simulink model "W2_Problem_4"  (R2020a)
settings: Solver=ode45  StartTime=0.0  StopTime=10.0  RelTol=1e-3
values from neighbouring files (symbols this model uses):
  b = 3.5077E-6    (= 3.5077e-06)    [W2_P4.m]    (also in W2_P4_DD.sldd = 3.5077E-6)
  J = 3.2284E-6    (= 3.2284e-06)    [W2_P4.m]    (also in W2_P4_DD.sldd = 3.2284E-6)
  K = 0.0274    [W2_P4.m]    (also in W2_P4_DD.sldd)
  Kd = Kd + 0.1    (= 0.15)    [W2_P4.m]    (also in W2_P4_DD.sldd = 0.44999999999999996)
  Ki = 500    [W2_P4.m]    (also in W2_P4_DD.sldd = 100.0)
  Kp = 21    [W2_P4.m]    (also in W2_P4_DD.sldd = 21.0)
  L = 2.75E-6    (= 2.75e-06)    [W2_P4.m]    (also in W2_P4_DD.sldd = 2.75E-6)
  R = 4    [W2_P4.m]    (also in W2_P4_DD.sldd = 4.0)
settings Model: Creator=user  LastModifiedBy=user

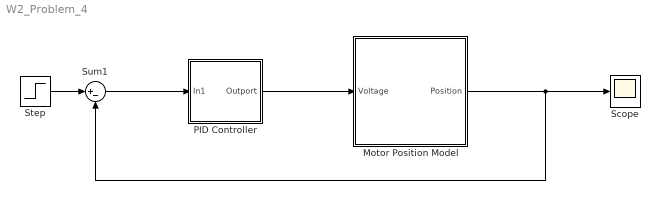
== system W2_Problem_4 ==
  Motor Position Model : Subsystem
  PID Controller : Subsystem
  Scope : Scope
  Step : Step  SampleTime=0
  Sum1 : Sum  Inputs=|+-
  wires:
  PID Controller/1(Outport) -> Motor Position Model/1(Voltage)
  Motor Position Model/1(Position) -> Scope/1, Sum1/2
  Sum1/1 -> PID Controller/1(In1)
  Step/1 -> Sum1/1

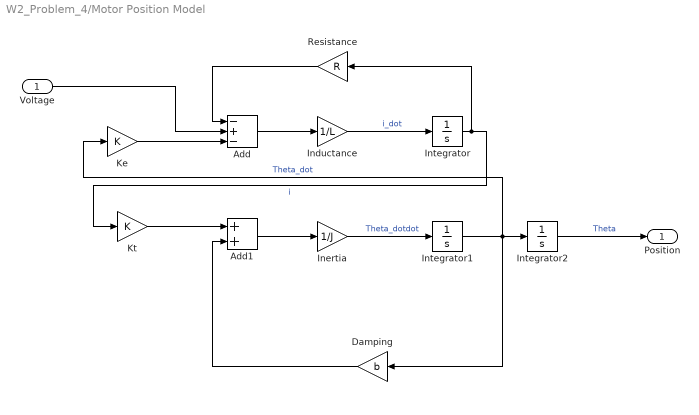
== system W2_Problem_4/Motor Position Model ==
  Voltage : Inport
  Add : Sum  Inputs=-+-
  Add1 : Sum
  Damping : Gain  Gain=b
  Inductance : Gain  Gain=1/L
  Inertia : Gain  Gain=1/J
  Integrator : Integrator
  Integrator1 : Integrator
  Integrator2 : Integrator
  Ke : Gain  Gain=K
  Kt : Gain  Gain=K
  Resistance : Gain  Gain=R
  Position : Outport
  wires:
  Inductance/1 -> Integrator/1  "i_dot"
  Resistance/1 -> Add/1
  Add/1 -> Inductance/1
  Integrator/1 -> Resistance/1, Kt/1  "i"
  Integrator1/1 -> Ke/1, Damping/1, Integrator2/1  "Theta_dot"
  Damping/1 -> Add1/2
  Add1/1 -> Inertia/1
  Ke/1 -> Add/3
  Inertia/1 -> Integrator1/1  "Theta_dotdot"
  Integrator2/1 -> Position/1  "Theta"
  Kt/1 -> Add1/1
  Voltage/1 -> Add/2

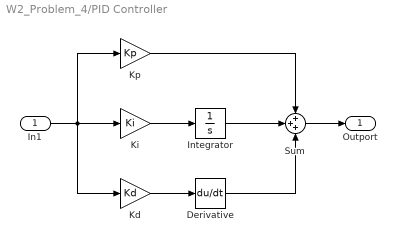
== system W2_Problem_4/PID Controller ==
  In1 : Inport
  Derivative : Derivative
  Integrator : Integrator
  Kd : Gain  Gain=Kd
  Ki : Gain  Gain=Ki
  Kp : Gain  Gain=Kp
  Sum : Sum  Inputs=+++
  Outport : Outport
  wires:
  Derivative/1 -> Sum/3
  Kd/1 -> Derivative/1
  Ki/1 -> Integrator/1
  In1/1 -> Kd/1, Kp/1, Ki/1
  Integrator/1 -> Sum/2
  Kp/1 -> Sum/1
  Sum/1 -> Outport/1
